simulink model "interview"  (R2021a)
settings: Solver=FixedStepAuto  StartTime=0.0  StopTime=1  FixedStep=0.1  RelTol=1e-3
libraries: simulink x1
settings Model: Creator=surya  LastModifiedBy=surya

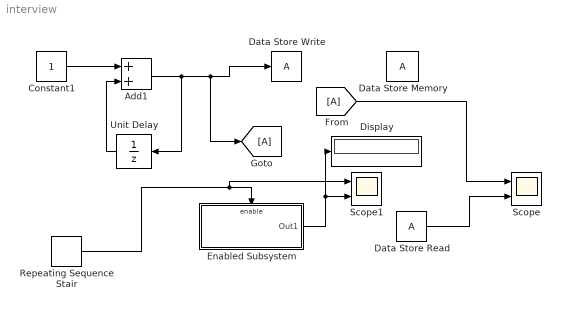
== system interview ==
  Add1 : Sum
  Constant1 : Constant
  Data Store Memory : DataStoreMemory  ReadBeforeWriteMsg=warning  WriteAfterWriteMsg=warning  WriteAfterReadMsg=warning  ShowAdditionalParam=off
  Data Store Read : DataStoreRead  IndexOptions=Index vector (dialog)  Indices=1  OutputSizes=1
  Data Store Write : DataStoreWrite  IndexOptions=Index vector (dialog)  Indices=1  OutputSizes=1
  Display : Display
  Enabled Subsystem : Subsystem  TreatAsAtomicUnit=on
  Repeating Sequence Stair : simulink/Sources/Repeating Sequence Stair  OutValues=[-0.1 -0.1 0 0 0 0 0 0 0.4 0.4].'  tsamp=-1  OutMin=[]  OutMax=[]  OutDataTypeStr=double  OutputDataTypeScalingMode=double  OutDataType=fixdt(0,8)  ConRadixGroup=Best Precision: Vector-wise  OutScaling=2^-12
  Scope : Scope  NumInputPorts=2
  Scope1 : Scope  NumInputPorts=2
  Unit Delay : UnitDelay  SampleTime=-1  HasFrameUpgradeWarning=on
  wires:
  Add1/1 -> Unit Delay/1, [A], Data Store Write/1
  Data Store Read/1 -> Scope/2
  Constant1/1 -> Add1/1
  Unit Delay/1 -> Add1/2
  [A] -> Scope/1
  Repeating Sequence Stair/1 -> Scope1/1, Enabled Subsystem/Enable
  Enabled Subsystem/1(Out1) -> Display/1, Scope1/2

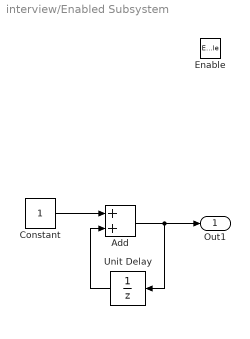
== system interview/Enabled Subsystem ==
  Enable : EnablePort
  Add : Sum
  Constant : Constant
  Unit Delay : UnitDelay  SampleTime=-1  HasFrameUpgradeWarning=on
  Out1 : Outport
  wires:
  Constant/1 -> Add/1
  Add/1 -> Unit Delay/1, Out1/1
  Unit Delay/1 -> Add/2
